simulink model "model5"  (R2022b)
settings: Solver=VariableStepAuto  StartTime=0.0  StopTime=10.0  RelTol=1e-3
values from neighbouring files (symbols this model uses):
  obj1 = [60, 45]    [init5.m]
  obj2 = [30, 25]    [init5.m]
  range = 100    [init5.m]
  thr = 5    [init5.m]
undefined symbols (not defined in the file or in its folder): K1, K2, K3, K4, K5, X01, X02, X03, X04, X05, X1d, X1d_dot, X2d, X2d_dot, X3d, X3d_dot, X4d, X4d_dot, X5d, X5d_dot
libraries: slctrlblks x1
settings Model: Creator=dorec  LastModifiedBy=dorec

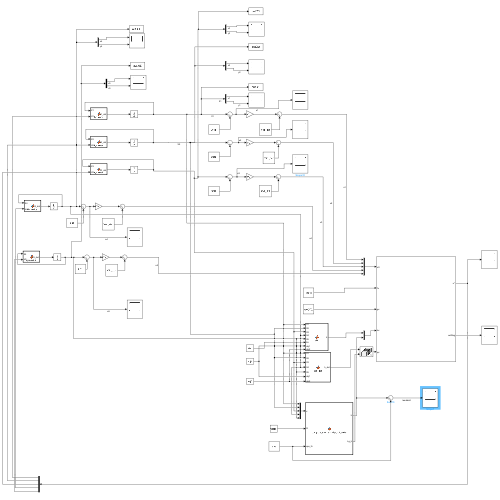
[thumbnail: Simulink's stored preview of the top-level diagram]
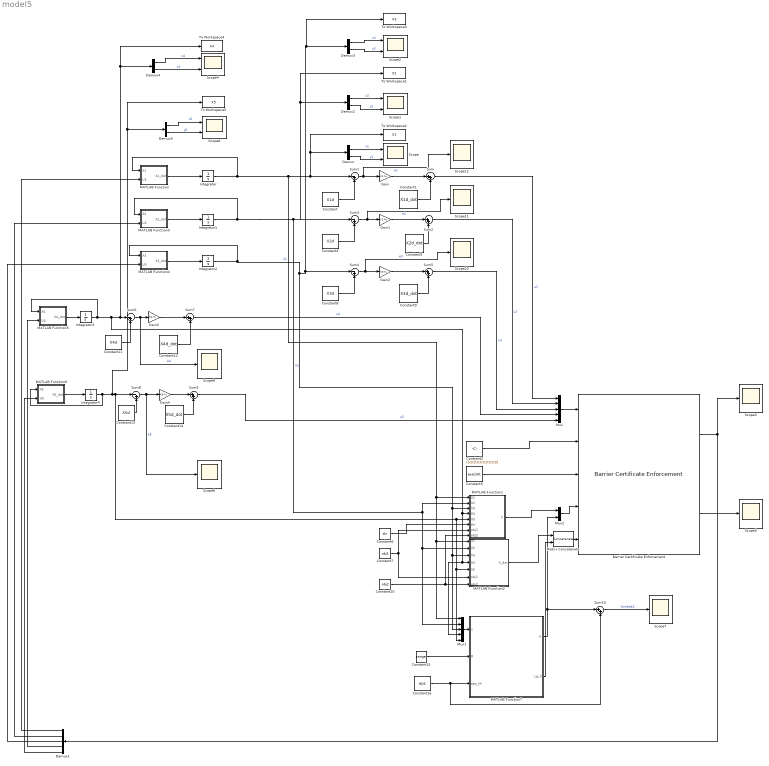
== system model5 ==
  Barrier Certificate Enforcement : slctrlblks/Barrier Certificate Enforcement  nx=10  nu=10  nc=21  gamma=10  beta=1  external_umax=off  external_umin=off  Ts=0.1  maxiter=200  tol=1e-6  output_exitflag=on
      settings: LibrarySourceBlock=slctrlblks/Constraint Control/Barrier Certificate Enforcement
  Constant : Constant  Value=X1d
  Constant1 : Constant  Value=X1d_dot
  Constant10 : Constant  Value=obj2
  Constant11 : Constant  Value=X4d
  Constant12 : Constant  Value=X4d_dot
  Constant13 : Constant  Value=X5d
  Constant14 : Constant  Value=X5d_dot
  Constant15 : Constant  Value=range
  Constant16 : Constant  Value=eps
  Constant2 : Constant  Value=[0;0;0;0;0;0;0;0;0;0]
  Constant3 : Constant  Value=eye(10);
  Constant4 : Constant  Value=X2d
  Constant5 : Constant  Value=X2d_dot
  Constant6 : Constant  Value=thr
  Constant7 : Constant  Value=obj1
  Constant8 : Constant  Value=X3d
  Constant9 : Constant  Value=X3d_dot
  Demux{,2..5} (5 alike) : Demux  Outputs=2
  Demux1 : Demux  Outputs=5
  Gain : Gain  Gain=K1  Multiplication=Matrix(K*u)
  Gain1 : Gain  Gain=K2  Multiplication=Matrix(K*u)
  Gain2 : Gain  Gain=K3  Multiplication=Matrix(K*u)
  Gain3 : Gain  Gain=K4  Multiplication=Matrix(K*u)
  Gain4 : Gain  Gain=K5  Multiplication=Matrix(K*u)
  Integrator : Integrator  InitialCondition=X01
  Integrator1 : Integrator  InitialCondition=X02
  Integrator2 : Integrator  InitialCondition=X03
  Integrator3 : Integrator  InitialCondition=X04
  Integrator4 : Integrator  InitialCondition=X05
  MATLAB Function : MATLAB Function  TreatAsAtomicUnit=on
  MATLAB Function1 : MATLAB Function  TreatAsAtomicUnit=on
  MATLAB Function2 : MATLAB Function  TreatAsAtomicUnit=on
  MATLAB Function3 : MATLAB Function  TreatAsAtomicUnit=on
  MATLAB Function4 : MATLAB Function  TreatAsAtomicUnit=on
  MATLAB Function5 : MATLAB Function  TreatAsAtomicUnit=on
  MATLAB Function6 : MATLAB Function  TreatAsAtomicUnit=on
  MATLAB Function7 : MATLAB Function  TreatAsAtomicUnit=on
  Matrix Concatenate : Concatenate  Mode=Multidimensional array
  Mux : Mux  Inputs=5
  Mux1 : Mux  Inputs=5
  Mux2 : Mux  Inputs=2
  Scope{,1..2,4,6} (5 alike) : Scope  NumInputPorts=2
  Scope{3,5,7..12} (8 alike) : Scope
  Sum{,2,5,7,9..10} (6 alike) : Sum  Inputs=|++
  Sum{1,3..4,6,8} (5 alike) : Sum  Inputs=|-+
  To Workspace1 : ToWorkspace  VariableName=X2  SaveFormat=Timeseries  SampleTime=-1
  To Workspace2 : ToWorkspace  VariableName=X1  SaveFormat=Timeseries  SampleTime=-1
  To Workspace3 : ToWorkspace  VariableName=X3  SaveFormat=Timeseries  SampleTime=-1
  To Workspace4 : ToWorkspace  VariableName=X4  SaveFormat=Timeseries  SampleTime=-1
  To Workspace5 : ToWorkspace  VariableName=X5  SaveFormat=Timeseries  SampleTime=-1
  wires:
  Integrator/1 -> Mux1/1, MATLAB Function2/1(X1), MATLAB Function1/1(X1), To Workspace2/1, Demux/1, Sum1/1, MATLAB Function/1(X1)  "X1"
  Sum1/1 -> Scope12/1, Gain/1  "e1"
  Constant/1 -> Sum1/2
  Gain/1 -> Sum/1
  Constant1/1 -> Sum/2
  Sum/1 -> Mux/1  "u1"
  MATLAB Function/1(X1_dot) -> Integrator/1
  Demux/1 -> Scope/1  "x1"
  Demux/2 -> Scope/2  "y1"
  MATLAB Function1/1(h) -> Mux2/1
  MATLAB Function2/1(h_dot) -> Matrix Concatenate/1
  Constant3/1 -> Barrier Certificate Enforcement/3
  Constant2/1 -> Barrier Certificate Enforcement/2
  Barrier Certificate Enforcement/1 -> Scope3/1, Demux1/1
  Constant5/1 -> Sum2/2
  Constant4/1 -> Sum3/2
  Gain1/1 -> Sum2/1
  Integrator1/1 -> MATLAB Function3/1(X2), To Workspace1/1, Demux2/1, Mux1/2, MATLAB Function2/2(X2), MATLAB Function1/2(X2), Sum3/1  "X2"
  MATLAB Function3/1(X2_dot) -> Integrator1/1
  Sum2/1 -> Mux/2  "u2"
  Mux/1 -> Barrier Certificate Enforcement/1
  Demux2/1 -> Scope1/1  "x2"
  Demux2/2 -> Scope1/2  "y2"
  Constant6/1 -> MATLAB Function1/6(thr)
  Constant7/1 -> MATLAB Function2/6(obj1), MATLAB Function1/7(obj1)
  MATLAB Function4/1(X3_dot) -> Integrator2/1
  Integrator2/1 -> Mux1/3, MATLAB Function2/3(X3), MATLAB Function1/3(X3), Demux3/1, To Workspace3/1, Sum4/1, MATLAB Function4/1(X3)
  Sum4/1 -> Scope10/1, Gain2/1  "e3"
  Constant8/1 -> Sum4/2
  Gain2/1 -> Sum5/1
  Constant9/1 -> Sum5/2
  Demux1/2 -> MATLAB Function3/2(U2)
  Demux3/2 -> Scope2/2  "y3"
  Demux3/1 -> Scope2/1  "x3"
  Constant10/1 -> MATLAB Function1/8(obj2), MATLAB Function2/7(obj2)
  MATLAB Function5/1(X4_dot) -> Integrator3/1
  Constant11/1 -> Sum6/2
  Sum6/1 -> Scope9/1, Gain3/1  "e4"
  Gain3/1 -> Sum7/1
  Constant12/1 -> Sum7/2
  Demux4/2 -> Scope4/2  "y4"
  Demux4/1 -> Scope4/1  "x4"
  Integrator3/1 -> MATLAB Function5/1(X4), Mux1/4, MATLAB Function2/4(X4), MATLAB Function1/4(X4), Demux4/1, To Workspace4/1, Sum6/1
  MATLAB Function6/1(X5_dot) -> Integrator4/1
  Integrator4/1 -> MATLAB Function6/1(X5), To Workspace5/1, Demux5/1, Sum8/1, Mux1/5, MATLAB Function2/5(X5), MATLAB Function1/5(X5)
  Constant13/1 -> Sum8/2
  Sum8/1 -> Scope8/1, Gain4/1  "e5"
  Gain4/1 -> Sum9/1
  Constant14/1 -> Sum9/2
  Demux1/5 -> MATLAB Function6/2(U5)
  Demux5/2 -> Scope6/2  "y5"
  Demux5/1 -> Scope6/1  "x5"
  Sum9/1 -> Mux/5  "u5"
  Sum5/1 -> Mux/3  "u3"
  Sum7/1 -> Mux/4  "u4"
  Demux1/1 -> MATLAB Function/2(U1)
  Demux1/3 -> MATLAB Function4/2(U3)
  Demux1/4 -> MATLAB Function5/2(U4)
  Constant15/1 -> MATLAB Function7/2(R)
  Constant16/1 -> Sum10/2, MATLAB Function7/3(eps_th)
  Mux1/1 -> MATLAB Function7/1(x)
  MATLAB Function7/1(h) -> Sum10/1, Mux2/2
  Matrix Concatenate/1 -> Barrier Certificate Enforcement/5
  MATLAB Function7/2(Lg_h) -> Matrix Concatenate/2
  Mux2/1 -> Barrier Certificate Enforcement/4
  Barrier Certificate Enforcement/2 -> Scope5/1
  Sum10/1 -> Scope7/1  "lambda2"
  Sum3/1 -> Scope11/1, Gain1/1  "e2"

== matlab function model5/MATLAB Function1 ==
  data: X1 input; X2 input; X3 input; X4 input; X5 input; thr input; h output; obj1 input; obj2 input
function h = cbf(X1, X2, X3, X4, X5, thr, obj1, obj2)
    h12 = norm(X1 - X2) - thr;
    h13 = norm(X1 - X3) - thr;
    h14 = norm(X1 - X4) - thr;
    h15 = norm(X1 - X5) - thr;

    h23 = norm(X2 - X3) - thr;
    h24 = norm(X2 - X4) - thr;
    h25 = norm(X2 - X5) - thr;

    h34 = norm(X3 - X4) - thr;
    h35 = norm(X3 - X5) - thr;

    h45 = norm(X4 - X5) - thr;


    h1o1 = norm(X1 - obj1) - thr;
    h2o1 = norm(X2 - obj1) - thr;
    h3o1 = norm(X3 - obj1) - thr;
    h4o1 = norm(X4 - obj1) - thr;
    h5o1 = norm(X5 - obj1) - thr;

    h1o2 = norm(X1 - obj2) - thr;
    h2o2 = norm(X2 - obj2) - thr;
    h3o2 = norm(X3 - obj2) - thr;
    h4o2 = norm(X4 - obj2) - thr;
    h5o2 = norm(X5 - obj2) - thr;


    h = [ h12; h13; h14; h15;
          h23; h24; h25;
          h34; h35;
          h45;
          h1o1; h2o1; h3o1; h4o1; h5o1;
          h1o2; h2o2; h3o2; h4o2; h5o2 ];
end

== matlab function model5/MATLAB Function ==
  data: X1 input; U1 input size=[2 1]; X1_dot output
function X1_dot = dynamics(X1,U1)

x1_dot = U1(1);
y1_dot = U1(2);

X1_dot = [x1_dot; y1_dot];

== matlab function model5/MATLAB Function2 ==
  data: X1 input; X2 input; X3 input; X4 input; X5 input; obj1 input; h_dot output; obj2 input
function h_dot = cbf_dot(X1, X2, X3, X4, X5, obj1, obj2)
    
    n12 = (X1 - X2)/norm(X1 - X2);
    n13 = (X1 - X3)/norm(X1 - X3);
    n14 = (X1 - X4)/norm(X1 - X4);
    n15 = (X1 - X5)/norm(X1 - X5);

    n23 = (X2 - X3)/norm(X2 - X3);
    n24 = (X2 - X4)/norm(X2 - X4);
    n25 = (X2 - X5)/norm(X2 - X5);

    n34 = (X3 - X4)/norm(X3 - X4);
    n35 = (X3 - X5)/norm(X3 - X5);

    n45 = (X4 - X5)/norm(X4 - X5);

    
    n1o1 = (X1 - obj1)/norm(X1 - obj1);
    n2o1 = (X2 - obj1)/norm(X2 - obj1);
    n3o1 = (X3 - obj1)/norm(X3 - obj1);
    n4o1 = (X4 - obj1)/norm(X4 - obj1);
    n5o1 = (X5 - obj1)/norm(X5 - obj1);

    
    n1o2 = (X1 - obj2)/norm(X1 - obj2);
    n2o2 = (X2 - obj2)/norm(X2 - obj2);
    n3o2 = (X3 - obj2)/norm(X3 - obj2);
    n4o2 = (X4 - obj2)/norm(X4 - obj2);
    n5o2 = (X5 - obj2)/norm(X5 - obj2);



    h_dot = [
        
        n12(1) n12(2)  -n12(1) -n12(2)   0 0   0 0   0 0; 
        n13(1) n13(2)   0 0  -n13(1) -n13(2)  0 0   0 0; 
        n14(1) n14(2)   0 0   0 0  -n14(1) -n14(2)  0 0; 
        n15(1) n15(2)   0 0   0 0   0 0  -n15(1) -n15(2); 

        0 0  n23(1) n23(2)  -n23(1) -n23(2)  0 0   0 0; 
        0 0  n24(1) n24(2)   0 0  -n24(1) -n24(2)  0 0; 
        0 0  n25(1) n25(2)   0 0   0 0  -n25(1) -n25(2); 

        0 0   0 0  n34(1) n34(2)  -n34(1) -n34(2)  0 0; 
        0 0   0 0  n35(1) n35(2)   0 0  -n35(1) -n35(2); 

        0 0   0 0   0 0  n45(1) n45(2)  -n45(1) -n45(2); 

        n1o1(1) n1o1(2)  0 0 0 0 0 0 0 0; 
        0 0  n2o1(1) n2o1(2)  0 0 0 0 0 0; 
        0 0  0 0  n3o1(1) n3o1(2)  0 0 0 0; 
        0 0  0 0  0 0  n4o1(1) n4o1(2)  0 0; 
        0 0  0 0  0 0  0 0  n5o1(1) n5o1(2); 

        n1o2(1) n1o2(2)  0 0 0 0 0 0 0 0;
        0 0  n2o2(1) n2o2(2)  0 0 0 0 0 0; 
        0 0  0 0  n3o2(1) n3o2(2)  0 0 0 0;
        0 0  0 0  0 0  n4o2(1) n4o2(2)  0 0;
        0 0  0 0  0 0  0 0  n5o2(1) n5o2(2); 
    ];
end

== matlab function model5/MATLAB Function3 ==
  data: X2 input; U2 input size=[2 1]; X2_dot output
function X2_dot = dynamics(X2,U2)

x2_dot = U2(1);
y2_dot = U2(2);

X2_dot = [x2_dot; y2_dot];

== matlab function model5/MATLAB Function4 ==
  data: X3 input; U3 input size=[2 1]; X3_dot output
function X3_dot = dynamics(X3,U3)

x3_dot = U3(1);
y3_dot = U3(2);

X3_dot = [x3_dot; y3_dot];

== matlab function model5/MATLAB Function5 ==
  data: X4 input; U4 input size=[2 1]; X4_dot output
function X4_dot = dynamics(X4,U4)

x4_dot = U4(1);
y4_dot = U4(2);

X4_dot = [x4_dot; y4_dot];

== matlab function model5/MATLAB Function6 ==
  data: X5 input; U5 input size=[2 1]; X5_dot output
function X5_dot = dynamics(X5,U5)

x5_dot = U5(1);
y5_dot = U5(2);

X5_dot = [x5_dot; y5_dot];

== matlab function model5/MATLAB Function7 ==
  data: x input; h output; R input; eps_th input; Lg_h output
function [h, Lg_h] = compute_connectivity_cbf_safe(x, R, eps_th)
% Simulink-friendly and robust computation of:
%  h = lambda2 - eps_th
%  Lg_h : 1 x (2N) gradient d lambda2 / d x
%  Lf_plus_alpha : scalar = phi * h  (Lf h = 0 for single-integrator)
%
% Inputs:
%  x       : 2N x 1 stacked positions [x1; y1; x2; y2; ...]
%  R       : communication radius
%  eps_th  : connectivity threshold epsilon
%  phi     : alpha gain (alpha(h) = phi*h)
%
% Notes:
%  - This uses a polynomial bump weight: a(d) = (1 - (d/R)^2)^3 for d<=R, 0 otherwise.
%  - Avoids division by zero and ensures numeric finiteness.

% Parameters
MIN_D = 1e-6;    % min distance to avoid division by zero
N = numel(x)/2;
pos = reshape(x,2,N)';   % N x 2

% Prealloc
A = zeros(N);
dmat = zeros(N);

% Build adjacency using polynomial bump (bounded and smooth)
for i=1:N-1
    xi = pos(i,:);
    for j=i+1:N
        xj = pos(j,:);
        rij = xi - xj;
        dij = sqrt( max( rij(1)^2 + rij(2)^2, 0 ) ); % non-negative
        dmat(i,j) = dij;
        dmat(j,i) = dij;
        if dij <= R
            % polynomial bump (smooth, bounded)
            t = (dij / R)^2;
            aij = (1 - t)^3;   % in [0,1]
        else
            aij = 0;
        end
        A(i,j) = aij;
        A(j,i) = aij;
    end
end

% Ensure numeric finiteness
A(~isfinite(A)) = 0;

% Laplacian
D = diag(sum(A,2));
L = D - A;

% compute eigenpairs (full eig) and force real (Simulink-safe)
[Vfull, Dfull] = eig(L);
Vfull = real(Vfull);
Dfull = real(Dfull);
dvals = diag(Dfull);
[dvals_s, idx] = sort(dvals);
% If network is disconnected, lambda2 may equal 0; still fine
if numel(dvals_s) >= 2
    lambda2 = dvals_s(2);
    v2 = Vfull(:, idx(2));
else
    % fallback: small network (N=1) or pathological - set lambda2=0
    lambda2 = 0;
    v2 = zeros(N,1);
end
v2 = real(v2);

h = lambda2 - eps_th;

% compute beta = d lambda2 / d x (1 x 2N)
beta = zeros(1, 2*N);

% Precompute constants for polynomial bump derivative:
% For a(d) = (1 - (d/R)^2)^3, da/dd = -6 * (1 - (d/R)^2)^2 * (d / R^2)
for i = 1:N
    grad_i = zeros(1,2); % d lambda2 / d xi
    xi = pos(i,:);
    for j = 1:N
        if j == i, continue; end
        dij = dmat(i,j);
        if dij <= R && dij > 0
            % safe derivative computation
            t = (dij / R)^2;
            % derivative da/dd
            dad_d = -6 * (1 - t)^2 * (dij / (R^2));
            % avoid dividing by zero
            inv_d = 1.0 / max(dij, MIN_D);
            % d a_ij / d x_i = dad_d * (x_i - x_j)/dij
            da_dx = dad_d * (pos(i,:) - pos(j,:)) * inv_d;
            weight = (v2(i) - v2(j))^2;
            % accumulate (strip any tiny imag parts)
            grad_i = grad_i + real(da_dx * weight);
        end
        % if dij == 0 -> skip contribution (or you may add small regularization)
    end
    beta( (2*(i-1)+1) : (2*i) ) = grad_i;
end

% Safety: ensure finite values
beta(~isfinite(beta)) = 0;

Lg_h = beta;

end
